simulink model "AdvancedLab"  (R2024b)
settings: Solver=ode45  StartTime=0.0  StopTime=10  RelTol=1e-3
settings Model: Creator=MOHAMED  LastModifiedBy=MOHAMED

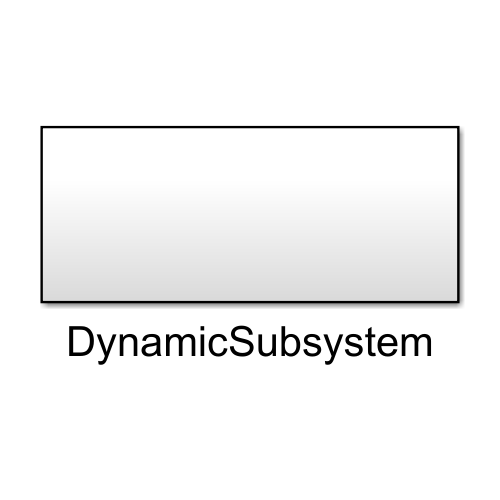
[thumbnail: Simulink's stored preview of the top-level diagram]
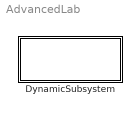
== system AdvancedLab ==
  DynamicSubsystem : Subsystem

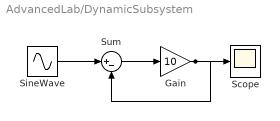
== system AdvancedLab/DynamicSubsystem ==
  Gain : Gain  Gain=10
  Scope : Scope
  SineWave : Sin  SampleTime=0
  Sum : Sum  Inputs=|+-
  wires:
  Gain/1 -> Sum/2, Scope/1
  SineWave/1 -> Sum/1
  Sum/1 -> Gain/1
